simulink model "task1_8"  (R2015b)
settings: Solver=ode45  StartTime=tstart  StopTime=tstop  RelTol=1e-3
values from neighbouring files (symbols this model uses):
  c = 0    [AnalyseSurgeSpeed.m]    (also in SurgeDynamicsTest.m; SurgeSpeedTest.m; analyse_dynamics.m; analyse_sway_dynamics.m)
  delta_max = deg2rad(25)    [SurgeSpeedTest.m]    (also in Yaw and Yaw-rate controller.mat = 0.436332312999; msfartoystyring.m = 0.436332312999)
  k_b0 = 0.009    [SurgeSpeedTest.m]    (also in Yaw and Yaw-rate controller.mat)
  K_d_u = 10    [run_task1_8.m]
  K_ff_u = 0.8    [run_task1_8.m]
  K_i_u = 1/400    (= 0.0025)    [run_task1_8.m]
  K_p_u = 3    [run_task1_8.m]
  kd_psi = 3    [SurgeSpeedTest.m]    (also in Yaw and Yaw-rate controller.mat)
  ki_psi = 2e-5    (= 2e-05)    [SurgeSpeedTest.m]    (also in Yaw and Yaw-rate controller.mat)
  kp_psi = 15e-3    (= 0.015)    [SurgeSpeedTest.m]    (also in Yaw and Yaw-rate controller.mat)
  n_c_max = 8.9    [AnalyseSpeedCharacteristis.m]    (also in AnalyseSpeedModel.m; AnalyseSurgeSpeed.m; Analyse_steadystate.m; Speed controller.mat)
  n_dot_max = 0.0436332312999    [Speed controller.mat]
  N_u = 1    [run_task1_8.m]
  psi0 = 0    [AnalyseSurgeSpeed.m]    (also in SurgeDynamicsTest.m; SurgeSpeedTest.m; analyse_dynamics.m; analyse_sway_dynamics.m)
  psi_s = deg2rad(45)    [SurgeSpeedTest.m]    (also in Yaw and Yaw-rate controller.mat = 0.785398163397)
  psi_t = 2000    [SurgeSpeedTest.m]    (also in Yaw and Yaw-rate controller.mat)
  r0 = 0    [AnalyseSurgeSpeed.m]    (also in SurgeDynamicsTest.m; SurgeSpeedTest.m; analyse_dynamics.m; analyse_sway_dynamics.m)
  tsamp = 10    [AnalyseSpeedCharacteristis.m]    (also in AnalyseSpeedModel.m; AnalyseSurgeSpeed.m; Analyse_steadystate.m; SurgeDynamicsTest.m)
  u_d = 5    [run_task1_8.m]
  v0 = [0.00001 0]'    [AnalyseSurgeSpeed.m]    (also in SurgeDynamicsTest.m = [1e-7 0]'; SurgeSpeedTest.m = [1e-7 0]'; analyse_dynamics.m = [1e-7 0]'; analyse_sway_dynamics.m = [6.63 0]')
  w_u = 0.011    [Speed controller.mat]
undefined symbols (not defined in the file or in its folder): msfartoystyring
undefined symbols (not defined in the file): p0
libraries: simulink x1
settings Model: ExtModeAutoUpdateStatusClock=off  Creator=christh  LastModifiedBy=Erik
settings DataIOCC: SaveFormat=Array  SignalLoggingSaveFormat=ModelDataLogs
settings OptimizationCC: ExpressionDepthLimit=2147483647  InitFltsAndDblsToZero=on
settings DebuggingCC: UnderspecifiedInitializationDetection=Classic  MergeDetectMultiDrivingBlocksExec=none  SolverPrmCheckMsg=warning  FcnCallInpInsideContextMsg=UseLocalSettings  StateNameClashWarn=warning
settings HardwareCC: ProdBitPerPointer=32  ProdLargestAtomicFloat=None  ProdIntDivRoundTo=Undefined  ProdEndianess=Unspecified  ProdWordSize=32  ProdHWDeviceType=32-bit Generic
settings GRTTargetCC: GeneratePreprocessorConditionals=Disable all  CombineOutputUpdateFcns=off  GRTInterface=on
settings ConfigComp: CovModelRefEnable=Off

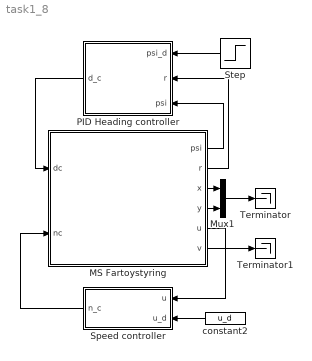
== system task1_8 ==
  MS Fartoystyring : Subsystem  mask(MS Fartoystyring for Assignment 3 G&C){x0=p0(1), y0=p0(2), u0=v0(1), v0=v0(2), psi0=psi0, r0=r0, c=c}
      mask prompts: x0 "x(t0) (m)"; y0 "y(t0) (m)"; u0 "u(t0) (m/s)"; v0 "v(t0) (m/s)"; psi0 "psi(t0) (rad)"; r0 "r(t0) (rad/s)"; c "current (0 or 1)"
      mask help:
      | Block corresponding to Figure 1 in the assignment text. Gives the response of the ship.
      |
      | The design speed of MS Fartoystyring is u=8.23 m/s.
      |
      | Input:
      | dc: commanded rudder (rad), dmax=25*pi/180
      | nc: commanded shaft speed (rad/s), nmax=85*2*pi/60
      |
      | Output:
      | x: north pos (m)
      | y: east pos (m)
      | u: surge (m/s)
      | v: sway (m/s)
      | psi: heading (rad)
      | r: yaw (rad/s)
      mask Help: Comments, bugs and help requests can be directed to the TA. Email on course website.
  Mux1 : Mux  Inputs=2
  PID Heading controller : Subsystem
  Speed controller : Subsystem
  Step : Step  Time=psi_t  After=psi_s  SampleTime=0
  Terminator : Terminator
  Terminator1 : Terminator
  constant2 : Constant  Value=u_d
  wires:
  MS Fartoystyring/1(psi) -> PID Heading controller/3(psi)
  MS Fartoystyring/2(r) -> PID Heading controller/2(r)
  constant2/1 -> Speed controller/2(u_d)
  Speed controller/1(n_c) -> MS Fartoystyring/2(nc)
  MS Fartoystyring/3(x) -> Mux1/1
  MS Fartoystyring/4(y) -> Mux1/2
  Mux1/1 -> Terminator/1
  MS Fartoystyring/6(v) -> Terminator1/1
  MS Fartoystyring/5(u) -> Speed controller/1(u)
  Step/1 -> PID Heading controller/1(psi_d)
  PID Heading controller/1(d_c) -> MS Fartoystyring/1(dc)

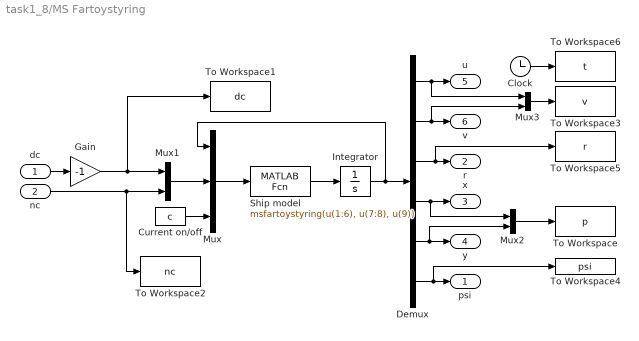
== system task1_8/MS Fartoystyring ==
  dc : Inport
  nc : Inport  Port=2
  Clock : Clock
  Current on/off : Constant  Value=c
  Demux : Demux  Outputs=6
  Gain : Gain  Gain=-1
  Integrator : Integrator  InitialCondition=[u0 v0 r0 x0 y0 psi0]'
  Mux : Mux  Inputs=3
  Mux1 : Mux  Inputs=2
  Mux2 : Mux  Inputs=2
  Mux3 : Mux  Inputs=2
  Ship model : MATLABFcn  MATLABFcn=msfartoystyring(u(1:6), u(7:8), u(9))  OutputDimensions=6
  To Workspace : ToWorkspace  VariableName=p  SampleTime=tsamp
  To Workspace1 : ToWorkspace  VariableName=dc  SampleTime=tsamp
  To Workspace2 : ToWorkspace  VariableName=nc  SampleTime=tsamp
  To Workspace3 : ToWorkspace  VariableName=v  SampleTime=tsamp
  To Workspace4 : ToWorkspace  VariableName=psi  SampleTime=tsamp
  To Workspace5 : ToWorkspace  VariableName=r  SampleTime=tsamp
  To Workspace6 : ToWorkspace  VariableName=t  SampleTime=tsamp
  psi : Outport
  r : Outport  Port=2
  x : Outport  Port=3
  y : Outport  Port=4
  u : Outport  Port=5
  v : Outport  Port=6
  wires:
  Integrator/1 -> Mux/1, Demux/1
  Mux1/1 -> Mux/2
  dc/1 -> Gain/1
  nc/1 -> Mux1/2, To Workspace2/1
  Demux/1 -> Mux3/1, u/1
  Demux/2 -> Mux3/2, v/1
  Demux/3 -> To Workspace5/1, r/1
  Demux/4 -> Mux2/1, x/1
  Demux/5 -> y/1, Mux2/2
  Demux/6 -> To Workspace4/1, psi/1
  Current on/off/1 -> Mux/3
  Ship model/1 -> Integrator/1
  Mux/1 -> Ship model/1
  Mux2/1 -> To Workspace/1
  Clock/1 -> To Workspace6/1
  Mux3/1 -> To Workspace3/1
  Gain/1 -> To Workspace1/1, Mux1/1

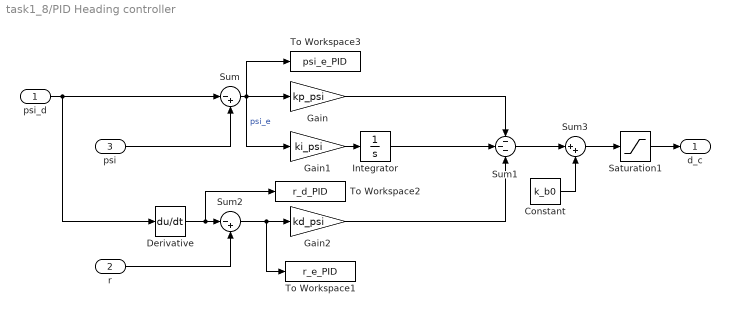
== system task1_8/PID Heading controller ==
  psi_d : Inport
  r : Inport  Port=2
  psi : Inport  Port=3
  Constant : Constant  Value=k_b0
  Derivative : Derivative
  Gain : Gain  Gain=kp_psi
  Gain1 : Gain  Gain=ki_psi
  Gain2 : Gain  Gain=kd_psi
  Integrator : Integrator
  Saturation1 : Saturate  UpperLimit=delta_max  LowerLimit=-delta_max
  Sum : Sum  Inputs=|-+
  Sum1 : Sum  Inputs=---
  Sum2 : Sum  Inputs=|-+
  Sum3 : Sum  Inputs=|++
  To Workspace1 : ToWorkspace  VariableName=r_e_PID  SampleTime=tsamp
  To Workspace2 : ToWorkspace  VariableName=r_d_PID  SampleTime=tsamp
  To Workspace3 : ToWorkspace  VariableName=psi_e_PID  SampleTime=tsamp
  d_c : Outport
  wires:
  psi_d/1 -> Derivative/1, Sum/1
  Saturation1/1 -> d_c/1
  Sum3/1 -> Saturation1/1
  psi/1 -> Sum/2
  Sum/1 -> Gain1/1, Gain/1, To Workspace3/1  "psi_e"
  Gain1/1 -> Integrator/1
  Gain/1 -> Sum1/1
  Integrator/1 -> Sum1/2
  Gain2/1 -> Sum1/3
  Sum1/1 -> Sum3/1
  Constant/1 -> Sum3/2
  Sum2/1 -> To Workspace1/1, Gain2/1
  r/1 -> Sum2/2
  Derivative/1 -> To Workspace2/1, Sum2/1

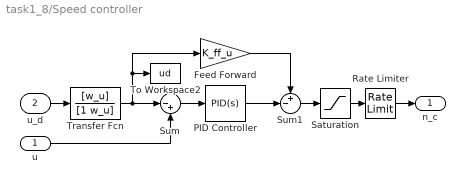
== system task1_8/Speed controller ==
  u : Inport
  u_d : Inport  Port=2
  Feed Forward : Gain  Gain=K_ff_u
  PID Controller : simulink/Continuous/PID Controller  Controller=PID  TimeDomain=Continuous-time  SampleTime=-1  IntegratorMethod=Forward Euler  FilterMethod=Forward Euler  Form=Parallel  UseFilter=on  ControllerParametersSource=internal  P=K_p_u  I=K_i_u  D=K_d_u  N=N_u  InitialConditionSource=internal  InitialConditionForIntegrator=0  InitialConditionForFilter=0  ExternalReset=none  LimitOutput=off  UpperSaturationLimit=inf  LowerSaturationLimit=-inf  LinearizeAsGain=on  AntiWindupMode=none  Kb=1  TrackingMode=off  Kt=1  PParamMin=[]  PParamMax=[]  IParamMin=[]  IParamMax=[]  DParamMin=[]  DParamMax=[]  NParamMin=[]  NParamMax=[]  KbParamMin=[]  KbParamMax=[]  KtParamMin=[]  KtParamMax=[]  POutMin=[]  POutMax=[]  IOutMin=[]  IOutMax=[]  DOutMin=[]  DOutMax=[]  NOutMin=[]  NOutMax=[]  KbOutMin=[]  KbOutMax=[]  KtOutMin=[]  KtOutMax=[]  IntegratorOutMin=[]  IntegratorOutMax=[]  FilterOutMin=[]  FilterOutMax=[]  SumOutMin=[]  SumOutMax=[]  SumI1OutMin=[]  SumI1OutMax=[]  SumI2OutMin=[]  SumI2OutMax=[]  SumI3OutMin=[]  SumI3OutMax=[]  SumDOutMin=[]  SumDOutMax=[]  SaturationOutMin=[]  SaturationOutMax=[]  IntegratorContinuousStateAttributes=''  IntegratorStateMustResolveToSignalObject=off  IntegratorRTWStateStorageClass=Auto  FilterContinuousStateAttributes=''  FilterStateMustResolveToSignalObject=off  FilterRTWStateStorageClass=Auto  DifferentiatorICPrevScaledInput=0  DifferentiatorOutMin=[]  DifferentiatorOutMax=[]
  Rate Limiter : RateLimiter  RisingSlewLimit=n_dot_max  FallingSlewLimit=-n_dot_max  SampleTimeMode=inherited
  Saturation : Saturate  UpperLimit=n_c_max  LowerLimit=-n_c_max
  Sum : Sum  Inputs=|-+
  Sum1 : Sum  Inputs=+-|
  To Workspace2 : ToWorkspace  VariableName=ud  SampleTime=tsamp
  Transfer Fcn : TransferFcn  Numerator=[w_u]  Denominator=[1 w_u]
  n_c : Outport
  wires:
  u_d/1 -> Transfer Fcn/1
  Sum1/1 -> Saturation/1
  Feed Forward/1 -> Sum1/1
  u/1 -> Sum/2
  Sum/1 -> PID Controller/1
  PID Controller/1 -> Sum1/2
  Saturation/1 -> Rate Limiter/1
  Transfer Fcn/1 -> Sum/1, Feed Forward/1, To Workspace2/1
  Rate Limiter/1 -> n_c/1
